simulink model "Exercicio_5_Vinicius"  (R2015a)
settings: Solver=ode45  StartTime=0.0  StopTime=400  FixedStep=Ts  RelTol=1e-3
values from neighbouring files (symbols this model uses):
  AA = [Ab1,zeros(length(Ab1),length(Ab2))             ;zeros(length(Ab2),length(Ab1)),Ab2]    [Exercicio_5_Vinicius_Alexandre.m]
  BB = [Bb1;Bb2]    [Exercicio_5_Vinicius_Alexandre.m]
  DD = [D1,zeros(md,nd);zeros(md,nd),D2]    [Exercicio_5_Vinicius_Alexandre.m]
  dd = [0.0 0.2 0 0.2]    [Exercicio_5_Vinicius_Alexandre.m]
  H = [H1,zeros(1,length(Ab1));zeros(1,length(Ab1)),H1]    [Exercicio_5_Vinicius_Alexandre.m]
  KE = K*E    [Exercicio_5_Vinicius_Alexandre.m]
  KF = K*F    [Exercicio_5_Vinicius_Alexandre.m]
  Kp = 1.0    (= 1)    [Exercicio_5_Vinicius_Alexandre.m]
  KR = KR+K(1:nest,j:j+nest-1)    [Exercicio_5_Vinicius_Alexandre.m]
  Ts = 0.03    [Exercicio_5_Vinicius_Alexandre.m]
undefined symbols (not defined in the file or in its folder): pp
libraries: cstblocks x1, simulink x1
settings Model: Creator=vinic  LastModifiedBy=vinic

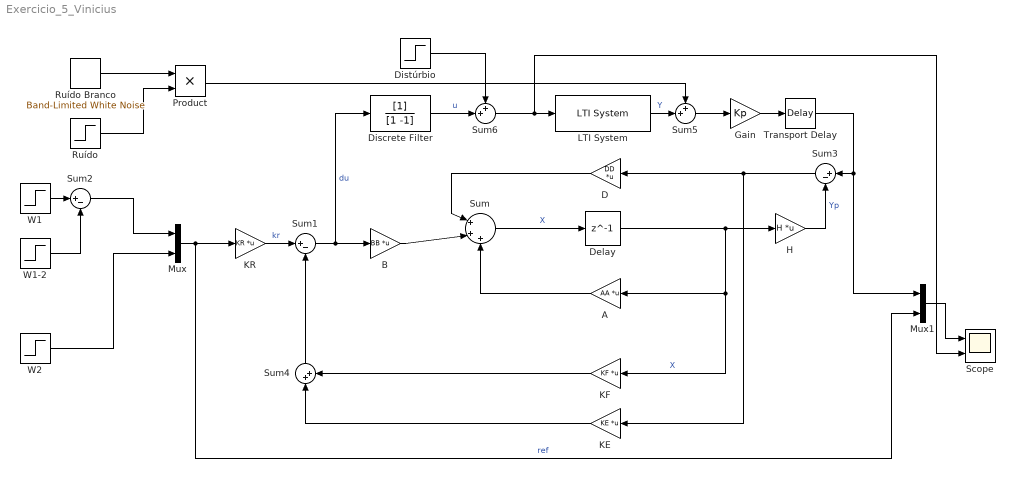
== system Exercicio_5_Vinicius ==
  A : Gain  Gain=AA  Multiplication=Matrix(K*u)
  B : Gain  Gain=BB  Multiplication=Matrix(K*u)
  D : Gain  Gain=DD  Multiplication=Matrix(K*u)
  Delay : Delay  DelayLength=1  SampleTime=Ts
  Discrete Filter : DiscreteFilter  Denominator=[1 -1]  SampleTime=Ts
  Distúrbio : Step  Time=2  After=.1  SampleTime=Ts
  Gain : Gain  Gain=Kp
  H : Gain  Gain=H  Multiplication=Matrix(K*u)
  KE : Gain  Gain=KE  Multiplication=Matrix(K*u)
  KF : Gain  Gain=KF  Multiplication=Matrix(K*u)
  KR : Gain  Gain=KR  Multiplication=Matrix(K*u)
  LTI System : cstblocks/LTI System  sys=Ct  IC=[]
  Mux : Mux  Inputs=2
  Mux1 : Mux  Inputs=2
  Product : Product
  Ruído : Step  Time=4  After=.2  SampleTime=Ts
  Ruído Branco : simulink/Sources/Band-Limited White Noise  Cov=Ts/5000  Ts=Ts/10  seed=[23341]
  Scope : Scope  NumInputPorts=2
      settings: YMin=0~-5  YMax=0.6~5  SaveName=simul
  Sum : Sum  Inputs=|+++
  Sum1 : Sum  Inputs=|+-
  Sum2 : Sum  Inputs=|+-
  Sum3 : Sum  Inputs=|+-
  Sum4 : Sum  Inputs=|++
  Sum5 : Sum  Inputs=++|
  Sum6 : Sum  Inputs=++|
  Transport Delay : TransportDelay  DelayTime=dd(pp)
  W1 : Step  Time=0  After=0.5  SampleTime=Ts
  W1-2 : Step  Time=1.5  After=0  SampleTime=Ts
  W2 : Step  Time=0  After=0.3  SampleTime=Ts
  wires:
  Sum/1 -> Delay/1  "X"
  Delay/1 -> KF/1, A/1, H/1  "X"
  A/1 -> Sum/3
  B/1 -> Sum/2
  D/1 -> Sum/1
  Sum3/1 -> KE/1, D/1
  Sum1/1 -> Discrete Filter/1, B/1  "du"
  H/1 -> Sum3/2  "Yp"
  KE/1 -> Sum4/1
  KF/1 -> Sum4/2
  Sum4/1 -> Sum1/2
  Mux/1 -> Mux1/2, KR/1  "ref"
  KR/1 -> Sum1/1  "kr"
  W2/1 -> Mux/2
  W1/1 -> Sum2/1
  Sum2/1 -> Mux/1
  W1-2/1 -> Sum2/2
  Mux1/1 -> Scope/1
  Gain/1 -> Transport Delay/1
  Transport Delay/1 -> Mux1/1, Sum3/1
  Ruído Branco/1 -> Product/1
  Product/1 -> Sum5/1
  Ruído/1 -> Product/2
  LTI System/1 -> Sum5/2  "Y"
  Sum5/1 -> Gain/1
  Sum6/1 -> Scope/2, LTI System/1
  Discrete Filter/1 -> Sum6/2  "u"
  Distúrbio/1 -> Sum6/1
